simulink model "Contr"  (R2023a)
settings: Solver=VariableStepAuto  StartTime=0.0  StopTime=300  RelTol=1e-3
values from neighbouring files (symbols this model uses):
  Ak = A-B*K    [Script_Dirigibile.m]
  x0_tilde = [x0(1)-xeq(1) x0(2)-xeq(2) x0(3)-xeq(3)]    [Script_Dirigibile.m]
  xeq = x_eq    [Script_Dirigibile.m]
  yeq = x_eq    [Script_Dirigibile.m]
undefined symbols (not defined in the file or in its folder): B
settings Model: Creator=giuco  LastModifiedBy=giuco

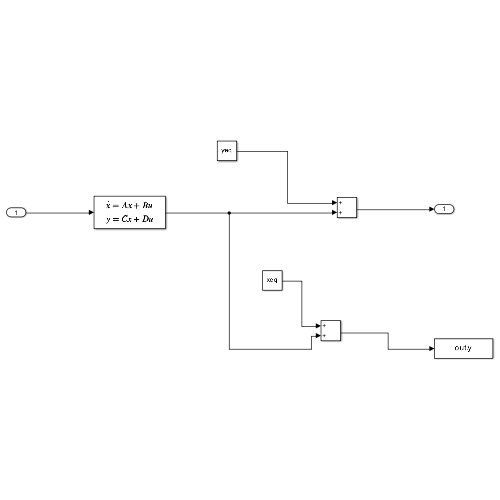
[thumbnail: Simulink's stored preview of the top-level diagram]
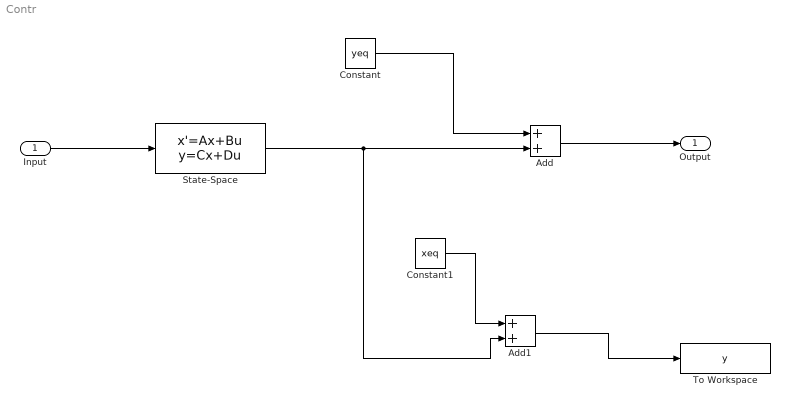
== system Contr ==
  Input : Inport
  Add : Sum
  Add1 : Sum
  Constant : Constant  Value=yeq
  Constant1 : Constant  Value=xeq
  State-Space : StateSpace  A=Ak  B=B  C=eye(3)  D=zeros(3,1)  InitialCondition=x0_tilde
  To Workspace : ToWorkspace  VariableName=y  SaveFormat=Timeseries  SampleTime=-1
  Output : Outport
  wires:
  Constant/1 -> Add/1
  Input/1 -> State-Space/1
  Add/1 -> Output/1
  State-Space/1 -> Add1/2, Add/2
  Constant1/1 -> Add1/1
  Add1/1 -> To Workspace/1
